simulink model "KociolPom1CvwCvg"  (R2025b)
settings: Solver=ode45  StartTime=0.0  StopTime=3000  MaxStep=1  RelTol=1e-3  AbsTol=1e-6
values from neighbouring files (symbols this model uses):
  czas_skok = 500    [KociolPom1CvwCvg_skrypt.m]
  dFg = 0*FgN    [KociolPom1CvwCvg_skrypt.m]
  dQk = 0.2* QkN    (= 400)    [KociolPom1CvwCvg_skrypt.m]
  dQt = 0    [KociolPom1CvwCvg_skrypt.m]
  dTzew = 0    [KociolPom1CvwCvg_skrypt.m]
  Fg0 = FgN    [KociolPom1CvwCvg_skrypt.m]
  Kcg = QgN/(TgpN-TwewN)    (= 40)    [KociolPom1CvwCvg_skrypt.m]
  Kcw = QgN/(TwewN-TzewN)    (= 50)    [KociolPom1CvwCvg_skrypt.m]
  Qk0 = QkN    (= 2000)    [KociolPom1CvwCvg_skrypt.m]
  Qt0 = 0    [KociolPom1CvwCvg_skrypt.m]
  Tgp0 = x0(2)    [KociolPom1CvwCvg_skrypt.m]
  Tkz0 = x0(3)    [KociolPom1CvwCvg_skrypt.m]
  Twew0 = x0(1)    [KociolPom1CvwCvg_skrypt.m]
  Tzew0 = TzewN+0    (= -20)    [KociolPom1CvwCvg_skrypt.m]
undefined symbols (not defined in the file or in its folder): cpw, Cvg, Cvk, Cvws, To
libraries: simulink x1
settings Model: ExtModeTrigMode=oneshot  ExtModeArmWhenConnect=off  Creator=ac  LastModifiedBy=jgzim
settings SolverCC: AutoScaleAbsTol=off  AlgebraicLoopSolver=TrustRegion
settings DataIOCC: SaveFormat=Array  SignalLoggingSaveFormat=ModelDataLogs  ReturnWorkspaceOutputs=off
settings OptimizationCC: BlockReduction=off  BooleanDataType=off  ExpressionDepthLimit=2147483647.0  LifeSpan=inf
settings DebuggingCC: SaveWithParameterizedLinksMsg=none  UnderspecifiedInitializationDetection=Classic  MergeDetectMultiDrivingBlocksExec=none  SignalResolutionControl=TryResolveAllWithWarning  MultiTaskDSMMsg=warning  MultiTaskCondExecSysMsg=none  FcnCallInpInsideContextMsg=warning  UnconnectedInputMsg=warning  UnconnectedOutputMsg=warning  UnconnectedLineMsg=warning  StateNameClashWarn=warning  SFUnexpectedBacktrackingDiag=warning  SFNoUnconditionalDefaultTransitionDiag=warning  SFExecutionAtInitializationDiag=none  ArithmeticOperatorsInVariantConditions=warning
settings HardwareCC: ProdBitPerPointer=32.0  ProdBitPerSizeT=32.0  ProdBitPerPtrDiffT=32.0  ProdLargestAtomicFloat=None  ProdIntDivRoundTo=Undefined  ProdEndianess=Unspecified  ProdWordSize=32.0  ProdHWDeviceType=32-bit Generic  TargetUnknown=on
settings ModelReferenceCC: PropagateSignalLabelsOutOfModel=off
settings SFSimCC: SimUseLocalCustomCode=off  CustomCodeUndefinedFunction=UseInterfaceOnly
settings RTWCC: RTWUseLocalCustomCode=off  GPUComputeCapability=3.5
settings CodeAppCC: StateflowObjectComments=on
settings GRTTargetCC: TargetLangStandard=C89/C90 (ANSI)  CombineOutputUpdateFcns=off  GRTInterface=on
settings ConfigComp: CovMetricSettings=dw  CovSaveCumulativeToWorkspaceVar=on  CovSaveSingleToWorkspaceVar=on  CovExternalEMLEnable=off

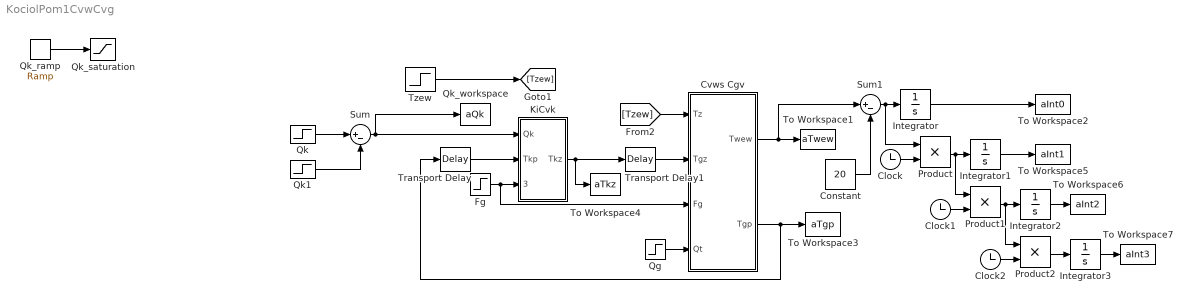
== system KociolPom1CvwCvg ==
  Clock : Clock
  Clock1 : Clock
  Clock2 : Clock
  Constant : Constant  Value=20
  Cvws Cgv : Subsystem
  Fg : Step  Time=czas_skok  Before=Fg0  After=Fg0+dFg  SampleTime=0
  Integrator{,1..3} (4 alike) : Integrator
  KiCvk : Subsystem  mask{cpw=cpw, Cvk=Cvk, Tkz0=Tkz0}
  Product : Product
  Product1 : Product
  Product2 : Product
  Qg : Step  Time=czas_skok  Before=Qt0  After=Qt0+dQt  SampleTime=0
  Qk : Step  Time=czas_skok  Before=Qk0  After=Qk0+dQk  SampleTime=0
  Qk1 : Step  Time=czas_skok + 0.0025  After=dQk  SampleTime=0
  Qk_ramp : simulink/Sources/Ramp  slope=0.007  start=czas_skok  InitialOutput=Qk0
  Qk_saturation : Saturate  UpperLimit=Qk0+dQk
  Qk_workspace : ToWorkspace  VariableName=aQk  SampleTime=-1
  Sum : Sum  Inputs=|+-
  Sum1 : Sum  Inputs=|+-
  To Workspace1 : ToWorkspace  VariableName=aTwew  SampleTime=-1
  To Workspace2 : ToWorkspace  VariableName=aInt0  SaveFormat=Timeseries  SampleTime=-1
  To Workspace3 : ToWorkspace  VariableName=aTgp  SampleTime=-1
  To Workspace4 : ToWorkspace  VariableName=aTkz  SampleTime=-1
  To Workspace5 : ToWorkspace  VariableName=aInt1  SaveFormat=Timeseries  SampleTime=-1
  To Workspace6 : ToWorkspace  VariableName=aInt2  SaveFormat=Timeseries  SampleTime=-1
  To Workspace7 : ToWorkspace  VariableName=aInt3  SaveFormat=Timeseries  SampleTime=-1
  Transport Delay : TransportDelay  DelayTime=To  InitialOutput=Tgp0
  Transport Delay1 : TransportDelay  DelayTime=To  InitialOutput=Tkz0
  Tzew : Step  Time=czas_skok  Before=Tzew0  After=Tzew0+dTzew  SampleTime=0
  wires:
  Fg/1 -> KiCvk/3(Fgm), Cvws Cgv/3(Fg)
  Transport Delay/1 -> KiCvk/2(Tkp)
  Cvws Cgv/1(Twew) -> Sum1/1, To Workspace1/1
  Cvws Cgv/2(Tgp) -> To Workspace3/1, Transport Delay/1
  Transport Delay1/1 -> Cvws Cgv/2(Tgz)
  [Tzew] -> Cvws Cgv/1(Tz)
  KiCvk/1(Tkz) -> Transport Delay1/1, To Workspace4/1
  Tzew/1 -> [Tzew]
  Qg/1 -> Cvws Cgv/4(Qt)
  Qk_ramp/1 -> Qk_saturation/1
  Qk/1 -> Sum/1
  Sum/1 -> Qk_workspace/1, KiCvk/1(Qk)
  Qk1/1 -> Sum/2
  Sum1/1 -> Product/1, Integrator/1
  Constant/1 -> Sum1/2
  Integrator/1 -> To Workspace2/1
  Clock/1 -> Product/2
  Product/1 -> Product1/1, Integrator1/1
  Integrator1/1 -> To Workspace5/1
  Clock1/1 -> Product1/2
  Product1/1 -> Product2/1, Integrator2/1
  Integrator2/1 -> To Workspace6/1
  Clock2/1 -> Product2/2
  Product2/1 -> Integrator3/1
  Integrator3/1 -> To Workspace7/1

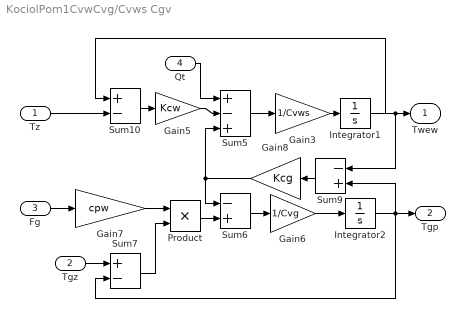
== system KociolPom1CvwCvg/Cvws Cgv ==
  Tz : Inport
  Tgz : Inport  Port=2
  Fg : Inport  Port=3
  Qt : Inport  Port=4
  Gain3 : Gain  Gain=1/Cvws  SaturateOnIntegerOverflow=on  OutDataTypeStr=Inherit: Same as input  ParamDataTypeStr=Inherit: Same as input
  Gain5 : Gain  Gain=Kcw  SaturateOnIntegerOverflow=on  OutDataTypeStr=Inherit: Same as input  ParamDataTypeStr=Inherit: Same as input
  Gain6 : Gain  Gain=1/Cvg  SaturateOnIntegerOverflow=on  OutDataTypeStr=Inherit: Same as input  ParamDataTypeStr=Inherit: Same as input
  Gain7 : Gain  Gain=cpw  SaturateOnIntegerOverflow=on  OutDataTypeStr=Inherit: Same as input  ParamDataTypeStr=Inherit: Same as input
  Gain8 : Gain  Gain=Kcg  SaturateOnIntegerOverflow=on  OutDataTypeStr=Inherit: Same as input  ParamDataTypeStr=Inherit: Same as input
  Integrator1 : Integrator  InitialCondition=Twew0
  Integrator2 : Integrator  InitialCondition=Tgp0
  Product : Product  InputSameDT=on  RndMeth=Zero  SaturateOnIntegerOverflow=on  OutDataTypeStr=Inherit: Same as first input
  Sum10 : Sum  Inputs=+-  InputSameDT=on  SaturateOnIntegerOverflow=on  OutDataTypeStr=Inherit: Same as first input
  Sum5 : Sum  Inputs=+-+  InputSameDT=on  SaturateOnIntegerOverflow=on  OutDataTypeStr=Inherit: Same as first input
  Sum6 : Sum  Inputs=-+  InputSameDT=on  SaturateOnIntegerOverflow=on  OutDataTypeStr=Inherit: Same as first input
  Sum7 : Sum  Inputs=+-  InputSameDT=on  SaturateOnIntegerOverflow=on  OutDataTypeStr=Inherit: Same as first input
  Sum9 : Sum  Inputs=-+  InputSameDT=on  SaturateOnIntegerOverflow=on  OutDataTypeStr=Inherit: Same as first input
  Twew : Outport
  Tgp : Outport  Port=2
  wires:
  Sum5/1 -> Gain3/1
  Sum6/1 -> Gain6/1
  Gain7/1 -> Product/1
  Sum7/1 -> Product/2
  Product/1 -> Sum6/2
  Gain6/1 -> Integrator2/1
  Integrator2/1 -> Sum7/2, Sum9/2, Tgp/1
  Sum9/1 -> Gain8/1
  Gain3/1 -> Integrator1/1
  Integrator1/1 -> Sum9/1, Sum10/1, Twew/1
  Sum10/1 -> Gain5/1
  Gain8/1 -> Sum6/1, Sum5/3
  Gain5/1 -> Sum5/2
  Qt/1 -> Sum5/1
  Fg/1 -> Gain7/1
  Tgz/1 -> Sum7/1
  Tz/1 -> Sum10/2

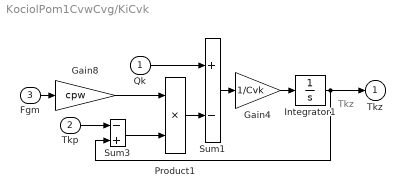
== system KociolPom1CvwCvg/KiCvk ==
  note: Tkz
  Qk : Inport
  Tkp : Inport  Port=2
  Fgm : Inport  Port=3
  Gain4 : Gain  Gain=1/Cvk  SaturateOnIntegerOverflow=on  OutDataTypeStr=Inherit: Same as input  ParamDataTypeStr=Inherit: Same as input
  Gain8 : Gain  Gain=cpw  SaturateOnIntegerOverflow=on  OutDataTypeStr=Inherit: Same as input  ParamDataTypeStr=Inherit: Same as input
  Integrator1 : Integrator  InitialCondition=Tkz0
  Product1 : Product  Inputs=**  InputSameDT=on  RndMeth=Zero  SaturateOnIntegerOverflow=on  OutDataTypeStr=Inherit: Same as first input
  Sum1 : Sum  Inputs=+-  InputSameDT=on  SaturateOnIntegerOverflow=on  OutDataTypeStr=Inherit: Same as first input
  Sum3 : Sum  Inputs=-+  InputSameDT=on  SaturateOnIntegerOverflow=on  OutDataTypeStr=Inherit: Same as first input
  Tkz : Outport
  wires:
  Tkp/1 -> Sum3/1
  Integrator1/1 -> Sum3/2, Tkz/1
  Product1/1 -> Sum1/2
  Sum1/1 -> Gain4/1
  Gain4/1 -> Integrator1/1
  Qk/1 -> Sum1/1
  Gain8/1 -> Product1/1
  Sum3/1 -> Product1/2
  Fgm/1 -> Gain8/1
